simulink model "robot3_model_dob_control"  (R2023b)
settings: Solver=FixedStepAuto  StartTime=0.0  StopTime=2*pi  RelTol=1e-3
undefined symbols (not defined in the file or in its folder): Cartesian_trajectory, Coriolis3, Dhat3, Dinv3, Forward_kin3, Gravity3
libraries: simulink x1, dspsrcs4 x1
settings Model: Creator=사용자  LastModifiedBy=rodel
settings SolverCC: ZeroCrossAlgorithm=Adaptive
settings DebuggingCC: IgnoredZcDiagnostic=none

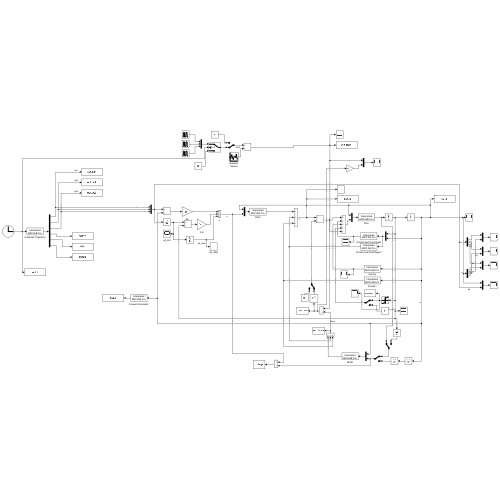
[thumbnail: Simulink's stored preview of the top-level diagram]
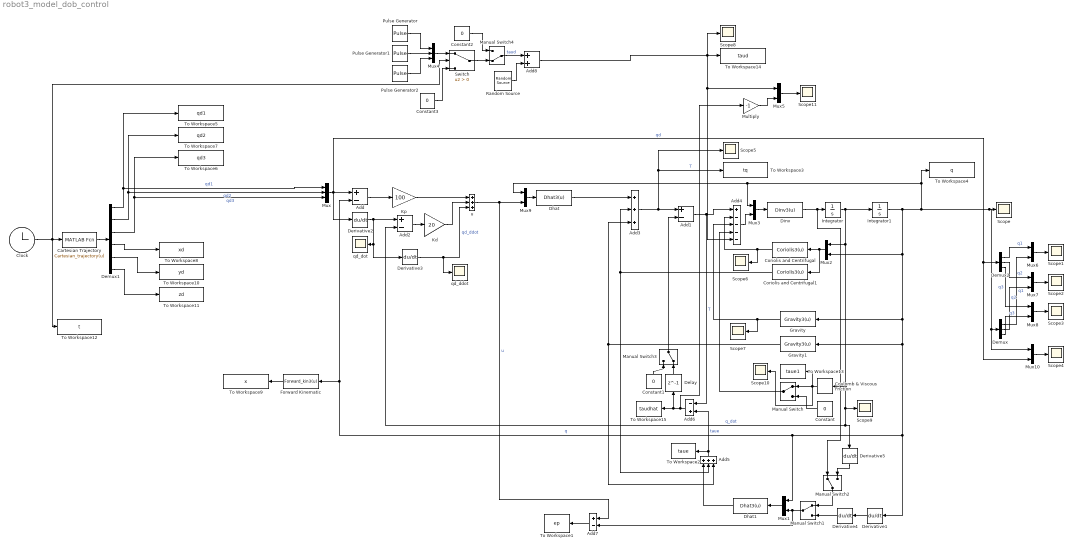
== system robot3_model_dob_control ==
  Add{,1..2,7} (4 alike) : Sum  Inputs=+-
  Add3 : Sum  Inputs=+++
  Add4 : Sum  Inputs=+----
  Add5 : Sum  Inputs=+++
  Add6 : Sum  Inputs=-+
  Add8 : Sum
  Cartesian Trajectory : MATLABFcn  MATLABFcn=Cartesian_trajectory(u)  OutputDimensions=6  Output1D=off
  Clock : Clock
  Constant{,1..3} (4 alike) : Constant  Value=0
  Coriolis and Centrifugal : MATLABFcn  MATLABFcn=Coriolis3(u)  OutputDimensions=3  Output1D=off
  Coriolis and Centrifugal1 : MATLABFcn  MATLABFcn=Coriolis3(u)  OutputDimensions=3  Output1D=off
  Coulomb & Viscous Friction : simulink/Discontinuities/Coulomb & Viscous Friction  offset=5  gain=3
  Delay : Delay  DelayLength=1  InitialCondition=0
  Demux : Demux  Outputs=3
  Demux1 : Demux  Outputs=6
  Demux2 : Demux  Outputs=3
  Derivative{1..5} (5 alike) : Derivative
  Dhat : MATLABFcn  MATLABFcn=Dhat3(u)  OutputDimensions=3  Output1D=off
  Dhat1 : MATLABFcn  MATLABFcn=Dhat3(u)  OutputDimensions=3  Output1D=off
  Dinv : MATLABFcn  MATLABFcn=Dinv3(u)  OutputDimensions=3  Output1D=off
  Forward Kinematic : MATLABFcn  MATLABFcn=Forward_kin3(u)  OutputDimensions=3  Output1D=off
  Gravity : MATLABFcn  MATLABFcn=Gravity3(u)  OutputDimensions=3  Output1D=off
  Gravity1 : MATLABFcn  MATLABFcn=Gravity3(u)  OutputDimensions=3  Output1D=off
  Integrator : Integrator  InitialCondition=[0;0;0];
  Integrator1 : Integrator  InitialCondition=[0.9587;0.7246;-1.1694]
  Kd : Gain  Gain=20
  Kp : Gain  Gain=100
  Manual Switch : ManualSwitch
  Manual Switch1 : ManualSwitch
  Manual Switch2 : ManualSwitch
  Manual Switch3 : ManualSwitch  CurrentSetting=0
  Manual Switch4 : ManualSwitch  CurrentSetting=0
  Multiply : Gain  Gain=-1
  Mux : Mux  Inputs=3
  Mux{1..3,5..10} (9 alike) : Mux  Inputs=2
  Mux4 : Mux  Inputs=3
  Pulse Generator : DiscretePulseGenerator  PulseType=Time based  Amplitude=10  PhaseDelay=2
  Pulse Generator1 : DiscretePulseGenerator  PulseType=Time based  Amplitude=10  PhaseDelay=3
  Pulse Generator2 : DiscretePulseGenerator  PulseType=Time based  Amplitude=10  PhaseDelay=1
  Random Source : dspsrcs4/Random Source  SrcType=Uniform  NormMethod=Ziggurat  CltLength=12  MinVal=0  MaxVal=5  MeanVal=0  VarVal=1  RepMode=Specify seed  rawSeed=345  IsInherit=off  SampMode=Discrete  SampTime=0.001  SampFrame=1  DataType=Double  OutComplex=Real  OutputFrames=off
  Scope{,1..11} (12 alike) : Scope
  Switch : Switch  Criteria=u2 > Threshold  SaturateOnIntegerOverflow=off  InputSameDT=off
  To Workspace1 : ToWorkspace  VariableName=ep  SaveFormat=Timeseries  SampleTime=0.001
  To Workspace10 : ToWorkspace  VariableName=yd  SampleTime=0.001
  To Workspace11 : ToWorkspace  VariableName=zd  SampleTime=0.001
  To Workspace12 : ToWorkspace  VariableName=t  SaveFormat=Timeseries  SampleTime=0.001
  To Workspace13 : ToWorkspace  VariableName=taue1  SaveFormat=Timeseries  SampleTime=0.001
  To Workspace14 : ToWorkspace  VariableName=taud  SaveFormat=Timeseries  SampleTime=0.001
  To Workspace15 : ToWorkspace  VariableName=taudhat  SaveFormat=Timeseries  SampleTime=0.001
  To Workspace2 : ToWorkspace  VariableName=taue  SaveFormat=Timeseries  SampleTime=0.001
  To Workspace3 : ToWorkspace  VariableName=tq  SaveFormat=Timeseries  SampleTime=0.001
  To Workspace4 : ToWorkspace  VariableName=q  SaveFormat=Timeseries  SampleTime=0.001
  To Workspace5 : ToWorkspace  VariableName=qd1  SaveFormat=Timeseries  SampleTime=0.001
  To Workspace6 : ToWorkspace  VariableName=qd3  SaveFormat=Timeseries  SampleTime=0.001
  To Workspace7 : ToWorkspace  VariableName=qd2  SaveFormat=Timeseries  SampleTime=0.001
  To Workspace8 : ToWorkspace  VariableName=xd  SampleTime=0.001
  To Workspace9 : ToWorkspace  VariableName=x  SampleTime=0.001
  qd_ddot : Scope
  qd_dot : Scope
  u : Sum  Inputs=+++
  wires:
  Mux/1 -> Derivative2/1, Mux10/2, Demux2/1, Add/1  "qd"
  Add2/1 -> Kd/1
  Kp/1 -> u/1
  Kd/1 -> u/2
  Add/1 -> Kp/1
  Dinv/1 -> Manual Switch2/1, Integrator/1
  Mux2/1 -> Coriolis and Centrifugal/1, Coriolis and Centrifugal1/1
  Integrator/1 -> Add2/2, Derivative5/1, Scope9/1, Coulomb & Viscous Friction/1, Mux2/1, Integrator1/1  "q_dot"
  Derivative3/1 -> qd_ddot/1, u/3  "qd_ddot"
  Mux9/1 -> Dhat/1
  Mux3/1 -> Dinv/1
  Add4/1 -> Mux3/2
  Dhat/1 -> Add3/1
  Coriolis and Centrifugal1/1 -> Add5/2, Add3/2
  Gravity1/1 -> Add5/3, Add3/3
  Coriolis and Centrifugal/1 -> Add4/2, Scope6/1
  Gravity/1 -> Add4/3, Scope7/1
  Constant/1 -> Manual Switch/2
  Manual Switch/1 -> Add4/4
  Coulomb & Viscous Friction/1 -> To Workspace13/1, Scope10/1, Manual Switch/1
  Derivative2/1 -> Derivative3/1, qd_dot/1, Add2/1
  Forward Kinematic/1 -> To Workspace9/1
  Demux1/5 -> To Workspace10/1
  Demux1/4 -> To Workspace8/1
  Demux1/3 -> To Workspace6/1, Mux/3  "qd3"
  Cartesian Trajectory/1 -> Demux1/1
  Demux1/1 -> To Workspace5/1, Mux/1  "qd1"
  Clock/1 -> Switch/2, Cartesian Trajectory/1, To Workspace12/1
  Demux1/6 -> To Workspace11/1
  Demux1/2 -> Mux/2, To Workspace7/1  "qd2"
  u/1 -> Mux9/2, Add7/1  "u"
  Add3/1 -> Scope5/1, To Workspace3/1, Add1/1  "T"
  Add1/1 -> Add6/1, Add4/1  "T"
  Derivative1/1 -> Derivative4/1
  Derivative4/1 -> Manual Switch1/2
  Derivative5/1 -> Manual Switch2/2
  Manual Switch2/1 -> Manual Switch1/1
  Manual Switch1/1 -> Add7/2, Mux1/2
  Mux1/1 -> Dhat1/1
  Add6/1 -> To Workspace15/1, Delay/1, Multiply/1
  Add5/1 -> To Workspace2/1, Add6/2  "taue"
  Delay/1 -> Manual Switch3/2
  Constant1/1 -> Manual Switch3/1
  Manual Switch3/1 -> Add1/2
  Dhat1/1 -> Add5/1
  Add7/1 -> To Workspace1/1
  Pulse Generator/1 -> Mux4/1
  Pulse Generator1/1 -> Mux4/2
  Pulse Generator2/1 -> Mux4/3
  Mux4/1 -> Switch/1
  Constant3/1 -> Switch/3
  Switch/1 -> Manual Switch4/2
  Constant2/1 -> Manual Switch4/1
  Demux/2 -> Mux7/2  "q2"
  Mux6/1 -> Scope1/1
  Mux7/1 -> Scope2/1
  Mux8/1 -> Scope3/1
  Integrator1/1 -> Mux2/2, Mux1/1, Forward Kinematic/1, Add/2, Derivative1/1, Gravity1/1, Gravity/1, Mux10/1, Demux/1, Scope/1, Mux3/1, Mux9/1, To Workspace4/1  "q"
  Demux/1 -> Mux6/2  "q1"
  Demux/3 -> Mux8/2  "q3"
  Mux10/1 -> Scope4/1
  Demux2/1 -> Mux6/1  "q1"
  Demux2/2 -> Mux7/1  "q2"
  Demux2/3 -> Mux8/1  "q3"
  Mux5/1 -> Scope11/1
  Multiply/1 -> Mux5/2
  Random Source/1 -> Add8/2
  Manual Switch4/1 -> Add8/1  "taud"
  Add8/1 -> Mux5/1, Add4/5, Scope8/1, To Workspace14/1
